simulink model "Inverse_Park"  (R2014b)
settings: Solver=ode45  StartTime=0.0  StopTime=10.0  RelTol=1e-3
settings Model: Creator=Eduardo Montilva  LastModifiedBy=Eduardo Montilva

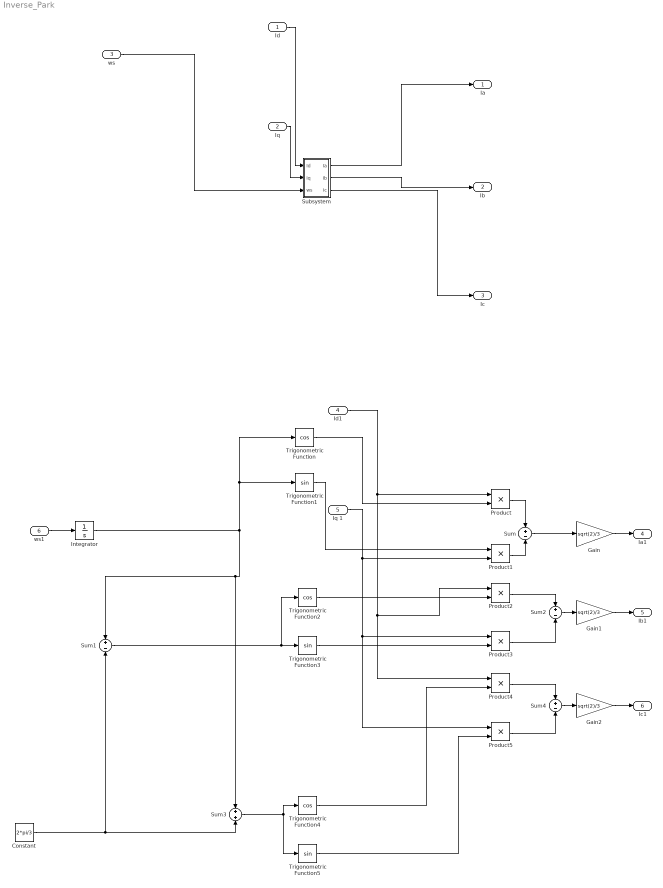
== system Inverse_Park ==
  Id : Inport
  "Iq " : Inport  Port=2
  ws : Inport  Port=3
  Id1 : Inport  Port=4
  Iq 1 : Inport  Port=5
  ws1 : Inport  Port=6
  Constant : Constant  Value=2*pi/3
  Gain : Gain  Gain=sqrt(2)/3
  Gain1 : Gain  Gain=sqrt(2)/3
  Gain2 : Gain  Gain=sqrt(2)/3
  Integrator : Integrator
  Product{,1..5} (6 alike) : Product
  Subsystem : Subsystem
  Sum{,1..2,4} (4 alike) : Sum  Inputs=+-
  Sum3 : Sum
  Trigonometric Function : Trigonometry  Operator=cos
  Trigonometric Function1 : Trigonometry
  Trigonometric Function2 : Trigonometry  Operator=cos
  Trigonometric Function3 : Trigonometry
  Trigonometric Function4 : Trigonometry  Operator=cos
  Trigonometric Function5 : Trigonometry
  Ia : Outport
  Ib : Outport  Port=2
  Ic : Outport  Port=3
  Ia1 : Outport  Port=4
  Ib1 : Outport  Port=5
  Ic1 : Outport  Port=6
  wires:
  Id/1 -> Subsystem/1(Id)
  "Iq "/1 -> Subsystem/2("Iq ")
  ws/1 -> Subsystem/3(ws)
  Subsystem/1(Ia) -> Ia/1
  Subsystem/2(Ib) -> Ib/1
  Subsystem/3(Ic) -> Ic/1
  Gain2/1 -> Ic1/1
  Product2/1 -> Sum2/1
  Product3/1 -> Sum2/2
  Sum3/1 -> Trigonometric Function4/1, Trigonometric Function5/1
  Id1/1 -> Product/1, Product4/1, Product2/1
  Trigonometric Function4/1 -> Product4/2
  Gain1/1 -> Ib1/1
  Sum1/1 -> Trigonometric Function2/1, Trigonometric Function3/1
  Constant/1 -> Sum1/2, Sum3/2
  Sum2/1 -> Gain1/1
  Trigonometric Function2/1 -> Product2/2
  Product/1 -> Sum/1
  Trigonometric Function/1 -> Product/2
  Integrator/1 -> Trigonometric Function1/1, Trigonometric Function/1, Sum3/1, Sum1/1
  ws1/1 -> Integrator/1
  Iq 1/1 -> Product5/1, Product3/1, Product1/2
  Gain/1 -> Ia1/1
  Trigonometric Function1/1 -> Product1/1
  Product1/1 -> Sum/2
  Sum/1 -> Gain/1
  Product5/1 -> Sum4/2
  Trigonometric Function5/1 -> Product5/2
  Product4/1 -> Sum4/1
  Sum4/1 -> Gain2/1
  Trigonometric Function3/1 -> Product3/2

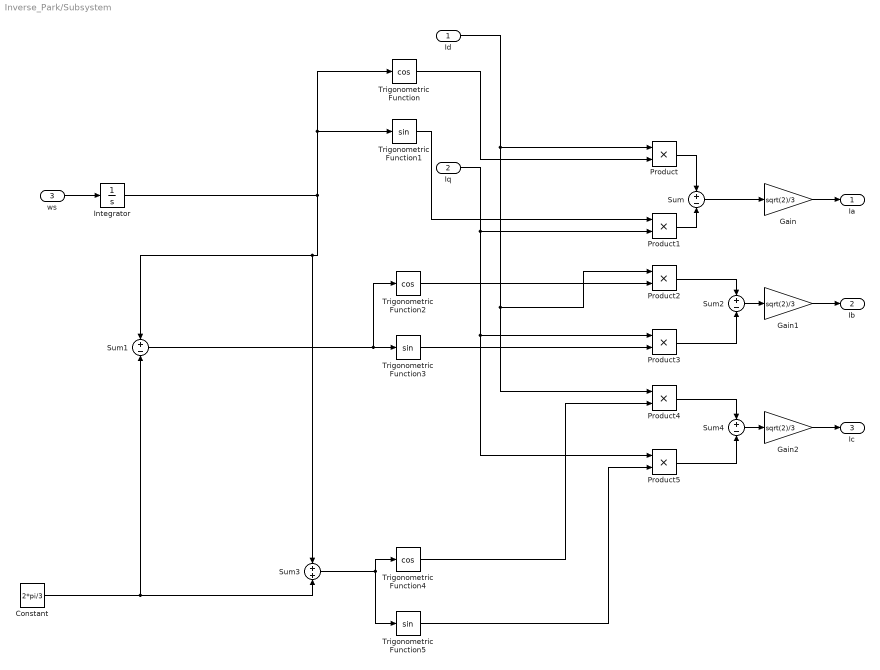
== system Inverse_Park/Subsystem ==
  Id : Inport
  "Iq " : Inport  Port=2
  ws : Inport  Port=3
  Constant : Constant  Value=2*pi/3
  Gain : Gain  Gain=sqrt(2)/3
  Gain1 : Gain  Gain=sqrt(2)/3
  Gain2 : Gain  Gain=sqrt(2)/3
  Integrator : Integrator
  Product{,1..5} (6 alike) : Product
  Sum{,1..2,4} (4 alike) : Sum  Inputs=+-
  Sum3 : Sum
  Trigonometric Function : Trigonometry  Operator=cos
  Trigonometric Function1 : Trigonometry
  Trigonometric Function2 : Trigonometry  Operator=cos
  Trigonometric Function3 : Trigonometry
  Trigonometric Function4 : Trigonometry  Operator=cos
  Trigonometric Function5 : Trigonometry
  Ia : Outport
  Ib : Outport  Port=2
  Ic : Outport  Port=3
  wires:
  Gain2/1 -> Ic/1
  Product2/1 -> Sum2/1
  Product3/1 -> Sum2/2
  Sum3/1 -> Trigonometric Function4/1, Trigonometric Function5/1
  Id/1 -> Product/1, Product4/1, Product2/1
  Trigonometric Function4/1 -> Product4/2
  Gain1/1 -> Ib/1
  Sum1/1 -> Trigonometric Function2/1, Trigonometric Function3/1
  Constant/1 -> Sum1/2, Sum3/2
  Sum2/1 -> Gain1/1
  Trigonometric Function2/1 -> Product2/2
  Product/1 -> Sum/1
  Trigonometric Function/1 -> Product/2
  Integrator/1 -> Trigonometric Function1/1, Trigonometric Function/1, Sum3/1, Sum1/1
  ws/1 -> Integrator/1
  "Iq "/1 -> Product5/1, Product3/1, Product1/2
  Gain/1 -> Ia/1
  Trigonometric Function1/1 -> Product1/1
  Product1/1 -> Sum/2
  Sum/1 -> Gain/1
  Product5/1 -> Sum4/2
  Trigonometric Function5/1 -> Product5/2
  Product4/1 -> Sum4/1
  Sum4/1 -> Gain2/1
  Trigonometric Function3/1 -> Product3/2
